simulink model "taskb"  (R2022a)
settings: Solver=VariableStepAuto  StartTime=0.0  StopTime=10.0  RelTol=1e-3  EnableMultiTasking=on
settings Model: Creator=DSP AND COMM LAB  LastModifiedBy=Zonularity
settings SolverCC: AlgebraicLoopSolver=TrustRegion
settings DataIOCC: ReturnWorkspaceOutputs=off
settings OptimizationCC: LifeSpan=inf
settings DebuggingCC: UnconnectedInputMsg=warning  UnconnectedOutputMsg=warning  UnconnectedLineMsg=warning  SFUnexpectedBacktrackingDiag=warning  SFNoUnconditionalDefaultTransitionDiag=warning  SFMachineParentedDataDiag=warning  ArithmeticOperatorsInVariantConditions=warning
settings SFSimCC: SimUseLocalCustomCode=off  CustomCodeUndefinedFunction=UseInterfaceOnly
settings RTWCC: RTWUseLocalCustomCode=off
settings CodeAppCC: StateflowObjectComments=on
settings GRTTargetCC: TargetLangStandard=C89/C90 (ANSI)
settings ConfigComp: CovMetricSettings=dw  CovSaveCumulativeToWorkspaceVar=on  CovSaveSingleToWorkspaceVar=on  CovExternalEMLEnable=off

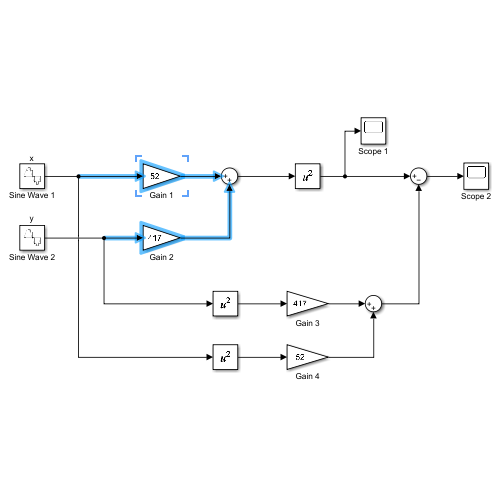
[thumbnail: Simulink's stored preview of the top-level diagram]
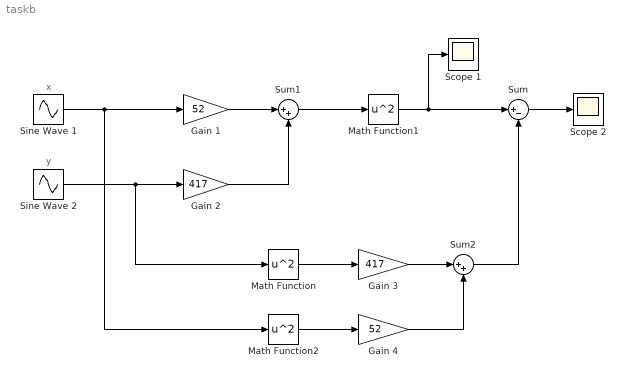
== system taskb ==
  note: y
  note: x
  Gain 1 : Gain  Gain=52
  Gain 2 : Gain  Gain=417
  Gain 3 : Gain  Gain=417
  Gain 4 : Gain  Gain=52
  Math Function : Math  Operator=square  SignedPower=on
  Math Function1 : Math  Operator=square  SignedPower=on
  Math Function2 : Math  Operator=square  SignedPower=on
  Scope 1 : Scope
  Scope 2 : Scope
  Sine Wave 1 : Sin  SampleTime=0.00001
  Sine Wave 2 : Sin  Frequency=2  SampleTime=0.00001
  Sum : Sum  Inputs=|+-
  Sum1 : Sum  Inputs=|++
  Sum2 : Sum  Inputs=|++
  wires:
  Sum1/1 -> Math Function1/1
  Math Function1/1 -> Sum/1, Scope 1/1
  Sum/1 -> Scope 2/1
  Math Function/1 -> Gain 3/1
  Sum2/1 -> Sum/2
  Sine Wave 1/1 -> Math Function2/1, Gain 1/1
  Sine Wave 2/1 -> Math Function/1, Gain 2/1
  Gain 1/1 -> Sum1/1
  Gain 2/1 -> Sum1/2
  Gain 3/1 -> Sum2/1
  Gain 4/1 -> Sum2/2
  Math Function2/1 -> Gain 4/1
